simulink model "MoveMissilesAttribute"  (R2022a)
settings: Solver=VariableStepAuto  StartTime=0.0  StopTime=60  RelTol=1e-3
libraries: robotlib x5, simulink_extras x1
settings Model: Creator=amani  LastModifiedBy=amani

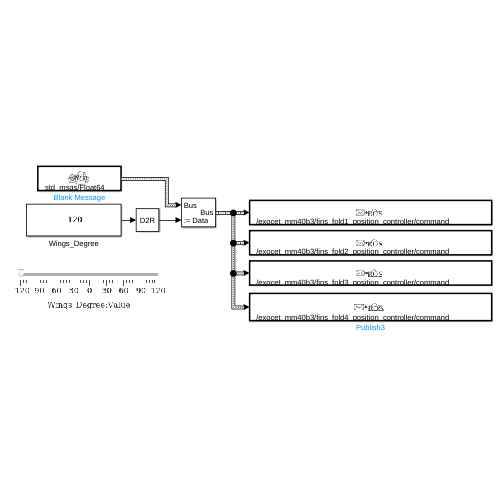
[thumbnail: Simulink's stored preview of the top-level diagram]
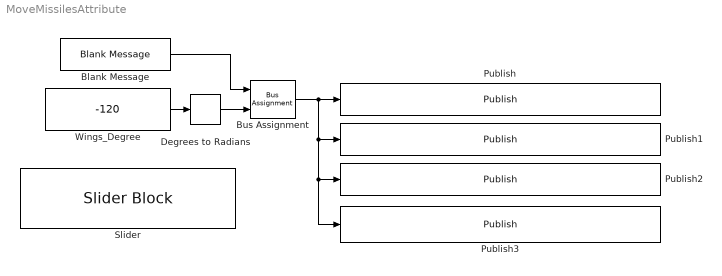
== system MoveMissilesAttribute ==
  Blank Message : robotlib/Blank Message  messageClass=Message  entityType=std_msgs/Float64  messageType=std_msgs/Float64  SampleTime=inf  legacyBusStruct=off
  Bus Assignment : BusAssignment  AssignedSignals=Data
  Degrees to Radians : simulink_extras/Transformations/Degrees to Radians
  Publish : robotlib/Publish  topicSource=Select from ROS network  topic=/exocet_mm40b3/fins_fold1_position_controller/command  messageType=std_msgs/Float64  legacyBusStruct=off  messageQueueLength=1
  Publish1 : robotlib/Publish  topicSource=Select from ROS network  topic=/exocet_mm40b3/fins_fold2_position_controller/command  messageType=std_msgs/Float64  legacyBusStruct=off  messageQueueLength=1
  Publish2 : robotlib/Publish  topicSource=Select from ROS network  topic=/exocet_mm40b3/fins_fold3_position_controller/command  messageType=std_msgs/Float64  legacyBusStruct=off  messageQueueLength=1
  Publish3 : robotlib/Publish  topicSource=Select from ROS network  topic=/exocet_mm40b3/fins_fold4_position_controller/command  messageType=std_msgs/Float64  legacyBusStruct=off  messageQueueLength=1
  Slider : SliderBlock  LabelPosition=Bottom  ScaleMin=-120  ScaleMax=120  TickInterval=30
  Wings_Degree : Constant  Value=-120
  wires:
  Wings_Degree/1 -> Degrees to Radians/1
  Bus Assignment/1 -> Publish3/1, Publish2/1, Publish1/1, Publish/1
  Blank Message/1 -> Bus Assignment/1
  Degrees to Radians/1 -> Bus Assignment/2
